simulink model "Mpc_SimMechanics_with_standing"  (R2017b)
settings: Solver=ode45  StartTime=0  StopTime=10  FixedStep=0.0005  EnableMultiTasking=on
InitFcn:
  | isSim = 1;
  | 
  | PreFunctions.CustomInitFcn_with_standing;
  | PreFunctions.simulationInitFcn_with_standing;
undefined symbols (not defined in the file): alpha_x, alpha_y, DiagnosticCodes, DynamicMatrixLibrary, motorPositions, motorVelocities, pelvisPosition, pelvisVelocity, sample_time, X, Y, Z
libraries: sm_lib x170, nesl_utility x75, Contact_Forces_Lib x6, ComponentLibrary x5, xpcrtudplib x2, slrtlib x1
(part 7 of 8)

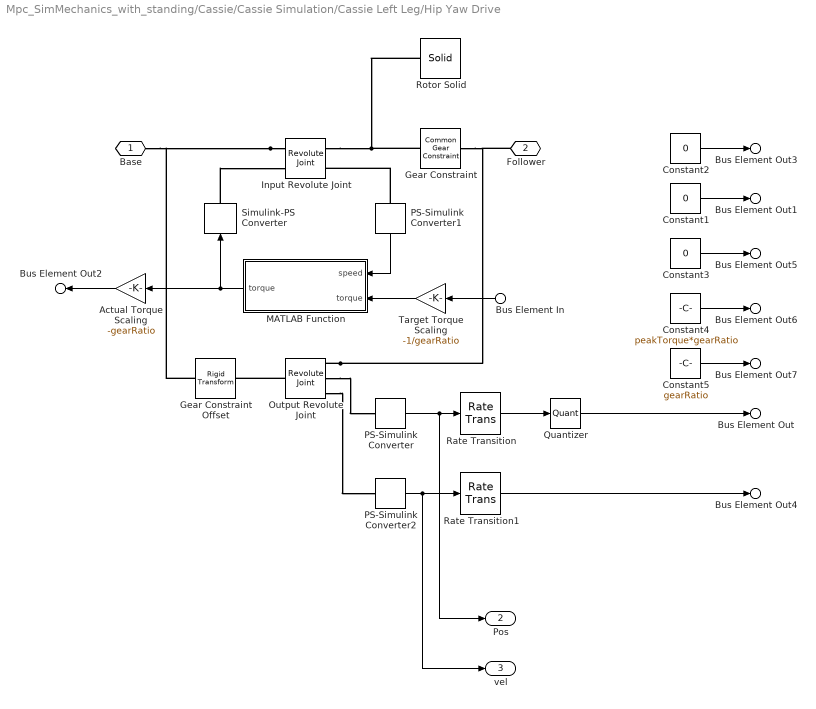
== system Mpc_SimMechanics_with_standing/Cassie/Cassie Simulation/Cassie Left Leg/Hip Yaw Drive ==
  Bus Element In : Inport  PortName=InBus  Element=torque
  Actual Torque Scaling : Gain  Gain=-gearRatio
  Constant1 : Constant  Value=0
  Constant2 : Constant  Value=0  OutDataTypeStr=uint16
  Constant3 : Constant  Value=0
  Constant4 : Constant  Value=peakTorque*gearRatio
  Constant5 : Constant  Value=gearRatio
  Gear Constraint : sm_lib/Gears and Couplings/Gears/Common Gear Constraint  GearType=External  SpecificationType=CenterDistanceRatio  CenterDistance=1e-6  CenterDistanceUnits=m  GearRatio=gearRatio  BaseGearRadius=10.0  BaseGearRadiusUnits=cm  FollGearRadius=10.0  FollGearRadiusUnits=cm  AssemblyGearRotation=Free
      settings: SourceProductName=Simscape Multibody  SourceProductBaseCode=MS
  Gear Constraint Offset : sm_lib/Frames and Transforms/Rigid Transform  TranslationMethod=StandardAxis  TranslationStandardOffset=1e-6  TranslationLengthUnit=m  TranslationStandardAxis=+Y  TranslationCartesianOffset=[0 0 0]  TranslationROffset=0  TranslationROffsetUnits=m  TranslationZOffset=0  TranslationZOffsetUnits=m  TranslationThetaOffset=0  TranslationThetaOffsetUnits=deg  RotationMethod=None  RotationAngleUnits=deg  RotationStandardAxis=+Z  RotationAngle=0.0  RotationArbitraryAxis=[0 0 1]  FollAlignAxisA=+X  BaseAlignAxisA=+Y  FollAlignAxisB=+Y  BaseAlignAxisB=+Z  RotationSequenceAxes=FollowerAxes  RotationSequence=XYX  RotationSequenceAngles=[0 0 0]  RotationSequenceAnglesUnits=deg  RotationMatrix=[1 0 0; 0 1 0; 0 0 1]
  Input Revolute Joint : sm_lib/Joints/Revolute Joint  SenseConstraintForce=off  SenseConstraintForceX=off  SenseConstraintForceY=off  SenseConstraintForceZ=off  SenseConstraintTorque=off  SenseConstraintTorqueX=off  SenseConstraintTorqueY=off  SenseConstraintTorqueZ=off  SenseTotalForce=off  SenseTotalForceX=off  SenseTotalForceY=off  SenseTotalForceZ=off  SenseTotalTorque=off  SenseTotalTorqueX=off  SenseTotalTorqueY=off  SenseTotalTorqueZ=off  CompositeWrenchDir=FollowerOnBase  CompositeWrenchFrame=BaseFrame  EquilibriumPosition=0  EquilibriumPositionUnits=rad  SpringStiffness=0  SpringStiffnessUnits=N*m/rad  DampingCoefficient=0  DampingCoefficientUnits=N*m/(rad/s)  TorqueActuationMode=InputTorque  MotionActuationMode=ComputedMotion  SensePosition=off  SenseVelocity=on  SenseAcceleration=off  SenseTorqueForce=off  PositionTargetSpecify=off  PositionTargetPriority=High  PositionTargetValue=0  PositionTargetValueUnits=deg  VelocityTargetSpecify=off  VelocityTargetPriority=High  VelocityTargetValue=0  VelocityTargetValueUnits=rad/s
  MATLAB Function : MATLAB Function  TreatAsAtomicUnit=on
  Output Revolute Joint : sm_lib/Joints/Revolute Joint  SenseConstraintForce=off  SenseConstraintForceX=off  SenseConstraintForceY=off  SenseConstraintForceZ=off  SenseConstraintTorque=off  SenseConstraintTorqueX=off  SenseConstraintTorqueY=off  SenseConstraintTorqueZ=off  SenseTotalForce=off  SenseTotalForceX=off  SenseTotalForceY=off  SenseTotalForceZ=off  SenseTotalTorque=off  SenseTotalTorqueX=off  SenseTotalTorqueY=off  SenseTotalTorqueZ=off  CompositeWrenchDir=FollowerOnBase  CompositeWrenchFrame=BaseFrame  EquilibriumPosition=0  EquilibriumPositionUnits=rad  SpringStiffness=0  SpringStiffnessUnits=N*m/rad  DampingCoefficient=1  DampingCoefficientUnits=N*m/(rad/s)  TorqueActuationMode=NoTorque  MotionActuationMode=ComputedMotion  SensePosition=on  SenseVelocity=on  SenseAcceleration=off  SenseTorqueForce=off  PositionTargetSpecify=on  PositionTargetPriority=High  PositionTargetValue=initialPosition  PositionTargetValueUnits=rad  VelocityTargetSpecify=on  VelocityTargetPriority=High  VelocityTargetValue=initialVelocity  VelocityTargetValueUnits=rad/s
  PS-Simulink Converter : nesl_utility/PS-Simulink Converter  PhysicalDomain=network_engine_domain  SubClassName=ps_output  LeftPortType=input  RightPortType=output  PseudoPeriodic=off  Frequencies=[]  Unit=rad  AffineConversion=off
  PS-Simulink Converter1 : nesl_utility/PS-Simulink Converter  PhysicalDomain=network_engine_domain  SubClassName=ps_output  LeftPortType=input  RightPortType=output  PseudoPeriodic=off  Frequencies=[]  Unit=rad/s  AffineConversion=off
  PS-Simulink Converter2 : nesl_utility/PS-Simulink Converter  PhysicalDomain=network_engine_domain  SubClassName=ps_output  LeftPortType=input  RightPortType=output  PseudoPeriodic=off  Frequencies=[]  Unit=rad/s  AffineConversion=off
  Quantizer : Quantizer  QuantizationInterval=(2*pi)/(encoderResolution*gearRatio)
  Rate Transition : RateTransition  Deterministic=off  InitialCondition=initialPosition  OutPortSampleTimeOpt=Inherit
  Rate Transition1 : RateTransition  Deterministic=off  InitialCondition=initialPosition  OutPortSampleTimeOpt=Inherit
  Rotor Solid : sm_lib/Body Elements/Solid  InertiaType=Custom  Mass=0  MassUnits=kg  CenterOfMass=[0; 0; 0]  CenterOfMassUnits=m  MomentsOfInertia=[0; 0; rotorInertia]  MomentsOfInertiaUnits=kg*m^2  ProductsOfInertia=[0; 0; 0]  ProductsOfInertiaUnits=kg*m^2  DensityBased=on  Density=1000  DensityUnits=kg/m^3  DoExposeReferenceFrame=on  SerializedFrames=<Frames/>  GraphicType=None  MarkerShape=Sphere  MarkerSize=10  GraphicVisPropType=SimpleVisualProperties  GraphicDiffuseColor=[0.5 0.5 0.5]  GraphicSpecularColor=[0.5 0.5 0.5 1.0]  GraphicAmbientColor=[0.15 0.15 0.15 1.0]  GraphicEmissiveColor=[0.0 0.0 0.0 1.0]  GraphicShininess=75  GraphicOpacity=1.0  GeometryShape=Cylinder  RectangleSize=[1 1]  RectangleSizeUnits=m  BrickDimensions=[1 1 1]  BrickDimensionUnits=m  CylinderRadius=1  CylinderRadiusUnits=m  CylinderLength=1  CylinderLengthUnits=m  SphereRadius=1  SphereRadiusUnits=m  EllipsoidRadii=[1 1 1]  EllipsoidRadiiUnits=m  ExtrusionCrossSection=[1 1; -1 1; -1 -1; 1 -1]  ExtrusionCrossSectionUnits=m  ExtrusionLength=1  ExtrusionLengthUnits=m  PolygonNumSides=3  PolygonOuterRadius=1  PolygonOuterRadiusUnits=m  ExtGeomFileType=STEP  ExtGeomFileUnits=m  RevolutionCrossSection=[1 1; 1 -1; 2 -1; 2 1]  RevolutionCrossSectionUnits=m  RevolutionExtent=Full  RevolutionAngle=180  RevolutionAngleUnits=deg
  Simulink-PS Converter : nesl_utility/Simulink-PS Converter  PhysicalDomain=network_engine_domain  SubClassName=ps_input  LeftPortType=input  RightPortType=output  PseudoPeriodic=off  Frequencies=[]  NoiseDistribution=none  NoiseParameters=[]  Unit=N*m  AffineConversion=off  FilteringAndDerivatives=zero  SimscapeFilterOrder=1  InputFilterTimeConstant=0.001  UdotUserProvided=1
  Target Torque Scaling : Gain  Gain=-1/gearRatio
  Base : PMIOPort  Port=1  Side=Left
  Follower : PMIOPort  Port=2  Side=Right
  Bus Element Out3 : Outport  PortName=OutBus  Element=statusWord
  Bus Element Out : Outport  PortName=OutBus  Element=position
  Bus Element Out4 : Outport  PortName=OutBus  Element=velocity
  Bus Element Out2 : Outport  PortName=OutBus  Element=torque
  Bus Element Out1 : Outport  PortName=OutBus  Element=driveTemperature
  Bus Element Out5 : Outport  PortName=OutBus  Element=dcLinkVoltage
  Bus Element Out6 : Outport  PortName=OutBus  Element=torqueLimit
  Bus Element Out7 : Outport  PortName=OutBus  Element=gearRatio
  Pos : Outport  Port=2
  vel : Outport  Port=3
  wires:
  PS-Simulink Converter2/1 -> vel/1, Rate Transition1/1
  Rate Transition1/1 -> Bus Element Out4/1
  Constant5/1 -> Bus Element Out7/1
  Actual Torque Scaling/1 -> Bus Element Out2/1
  Constant4/1 -> Bus Element Out6/1
  Constant3/1 -> Bus Element Out5/1
  Constant1/1 -> Bus Element Out1/1
  Constant2/1 -> Bus Element Out3/1
  Target Torque Scaling/1 -> MATLAB Function/2("torque ")
  PS-Simulink Converter1/1 -> MATLAB Function/1(speed)
  MATLAB Function/1(torque) -> Simulink-PS Converter/1, Actual Torque Scaling/1
  Bus Element In/1 -> Target Torque Scaling/1
  Quantizer/1 -> Bus Element Out/1
  PS-Simulink Converter/1 -> Pos/1, Rate Transition/1
  Rate Transition/1 -> Quantizer/1
  connections:
  Output Revolute Joint/RConn3 -- PS-Simulink Converter2/LConn1
  Input Revolute Joint/LConn1 -- Base/RConn1 -- Gear Constraint Offset/LConn1
  Simulink-PS Converter/RConn1 -- Input Revolute Joint/LConn2
  PS-Simulink Converter1/LConn1 -- Input Revolute Joint/RConn2
  Rotor Solid/RConn1 -- Gear Constraint/LConn1 -- Input Revolute Joint/RConn1
  Output Revolute Joint/RConn1 -- Follower/RConn1 -- Gear Constraint/RConn1
  Output Revolute Joint/LConn1 -- Gear Constraint Offset/RConn1
  Output Revolute Joint/RConn2 -- PS-Simulink Converter/LConn1

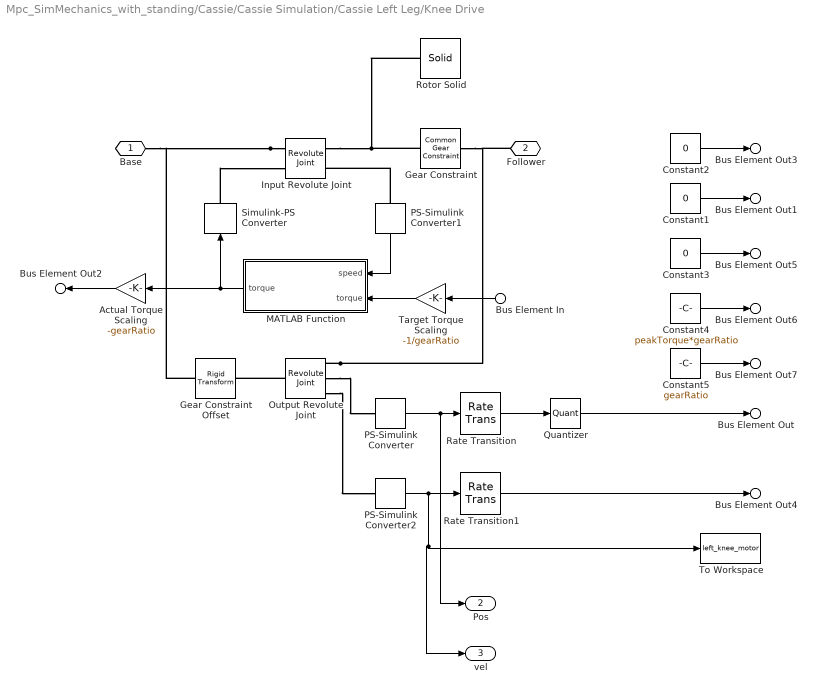
== system Mpc_SimMechanics_with_standing/Cassie/Cassie Simulation/Cassie Left Leg/Knee Drive ==
  Bus Element In : Inport  PortName=InBus  Element=torque
  Actual Torque Scaling : Gain  Gain=-gearRatio
  Constant1 : Constant  Value=0
  Constant2 : Constant  Value=0  OutDataTypeStr=uint16
  Constant3 : Constant  Value=0
  Constant4 : Constant  Value=peakTorque*gearRatio
  Constant5 : Constant  Value=gearRatio
  Gear Constraint : sm_lib/Gears and Couplings/Gears/Common Gear Constraint  GearType=External  SpecificationType=CenterDistanceRatio  CenterDistance=1e-6  CenterDistanceUnits=m  GearRatio=gearRatio  BaseGearRadius=10.0  BaseGearRadiusUnits=cm  FollGearRadius=10.0  FollGearRadiusUnits=cm  AssemblyGearRotation=Free
      settings: SourceProductName=Simscape Multibody  SourceProductBaseCode=MS
  Gear Constraint Offset : sm_lib/Frames and Transforms/Rigid Transform  TranslationMethod=StandardAxis  TranslationStandardOffset=1e-6  TranslationLengthUnit=m  TranslationStandardAxis=+Y  TranslationCartesianOffset=[0 0 0]  TranslationROffset=0  TranslationROffsetUnits=m  TranslationZOffset=0  TranslationZOffsetUnits=m  TranslationThetaOffset=0  TranslationThetaOffsetUnits=deg  RotationMethod=None  RotationAngleUnits=deg  RotationStandardAxis=+Z  RotationAngle=0.0  RotationArbitraryAxis=[0 0 1]  FollAlignAxisA=+X  BaseAlignAxisA=+Y  FollAlignAxisB=+Y  BaseAlignAxisB=+Z  RotationSequenceAxes=FollowerAxes  RotationSequence=XYX  RotationSequenceAngles=[0 0 0]  RotationSequenceAnglesUnits=deg  RotationMatrix=[1 0 0; 0 1 0; 0 0 1]
  Input Revolute Joint : sm_lib/Joints/Revolute Joint  SenseConstraintForce=off  SenseConstraintForceX=off  SenseConstraintForceY=off  SenseConstraintForceZ=off  SenseConstraintTorque=off  SenseConstraintTorqueX=off  SenseConstraintTorqueY=off  SenseConstraintTorqueZ=off  SenseTotalForce=off  SenseTotalForceX=off  SenseTotalForceY=off  SenseTotalForceZ=off  SenseTotalTorque=off  SenseTotalTorqueX=off  SenseTotalTorqueY=off  SenseTotalTorqueZ=off  CompositeWrenchDir=FollowerOnBase  CompositeWrenchFrame=BaseFrame  EquilibriumPosition=0  EquilibriumPositionUnits=rad  SpringStiffness=0  SpringStiffnessUnits=N*m/rad  DampingCoefficient=0  DampingCoefficientUnits=N*m/(rad/s)  TorqueActuationMode=InputTorque  MotionActuationMode=ComputedMotion  SensePosition=off  SenseVelocity=on  SenseAcceleration=off  SenseTorqueForce=off  PositionTargetSpecify=off  PositionTargetPriority=High  PositionTargetValue=0  PositionTargetValueUnits=deg  VelocityTargetSpecify=off  VelocityTargetPriority=High  VelocityTargetValue=0  VelocityTargetValueUnits=rad/s
  MATLAB Function : MATLAB Function  TreatAsAtomicUnit=on
  Output Revolute Joint : sm_lib/Joints/Revolute Joint  SenseConstraintForce=off  SenseConstraintForceX=off  SenseConstraintForceY=off  SenseConstraintForceZ=off  SenseConstraintTorque=off  SenseConstraintTorqueX=off  SenseConstraintTorqueY=off  SenseConstraintTorqueZ=off  SenseTotalForce=off  SenseTotalForceX=off  SenseTotalForceY=off  SenseTotalForceZ=off  SenseTotalTorque=off  SenseTotalTorqueX=off  SenseTotalTorqueY=off  SenseTotalTorqueZ=off  CompositeWrenchDir=FollowerOnBase  CompositeWrenchFrame=BaseFrame  EquilibriumPosition=0  EquilibriumPositionUnits=rad  SpringStiffness=0  SpringStiffnessUnits=N*m/rad  DampingCoefficient=1  DampingCoefficientUnits=N*m/(rad/s)  TorqueActuationMode=NoTorque  MotionActuationMode=ComputedMotion  SensePosition=on  SenseVelocity=on  SenseAcceleration=off  SenseTorqueForce=off  PositionTargetSpecify=on  PositionTargetPriority=High  PositionTargetValue=initialPosition  PositionTargetValueUnits=rad  VelocityTargetSpecify=on  VelocityTargetPriority=High  VelocityTargetValue=initialVelocity  VelocityTargetValueUnits=rad/s
  PS-Simulink Converter : nesl_utility/PS-Simulink Converter  PhysicalDomain=network_engine_domain  SubClassName=ps_output  LeftPortType=input  RightPortType=output  PseudoPeriodic=off  Frequencies=[]  Unit=rad  AffineConversion=off
  PS-Simulink Converter1 : nesl_utility/PS-Simulink Converter  PhysicalDomain=network_engine_domain  SubClassName=ps_output  LeftPortType=input  RightPortType=output  PseudoPeriodic=off  Frequencies=[]  Unit=rad/s  AffineConversion=off
  PS-Simulink Converter2 : nesl_utility/PS-Simulink Converter  PhysicalDomain=network_engine_domain  SubClassName=ps_output  LeftPortType=input  RightPortType=output  PseudoPeriodic=off  Frequencies=[]  Unit=rad/s  AffineConversion=off
  Quantizer : Quantizer  QuantizationInterval=(2*pi)/(encoderResolution*gearRatio)
  Rate Transition : RateTransition  Deterministic=off  InitialCondition=initialPosition  OutPortSampleTimeOpt=Inherit
  Rate Transition1 : RateTransition  Deterministic=off  InitialCondition=initialPosition  OutPortSampleTimeOpt=Inherit
  Rotor Solid : sm_lib/Body Elements/Solid  InertiaType=Custom  Mass=0  MassUnits=kg  CenterOfMass=[0; 0; 0]  CenterOfMassUnits=m  MomentsOfInertia=[0; 0; rotorInertia]  MomentsOfInertiaUnits=kg*m^2  ProductsOfInertia=[0; 0; 0]  ProductsOfInertiaUnits=kg*m^2  DensityBased=on  Density=1000  DensityUnits=kg/m^3  DoExposeReferenceFrame=on  SerializedFrames=<Frames/>  GraphicType=None  MarkerShape=Sphere  MarkerSize=10  GraphicVisPropType=SimpleVisualProperties  GraphicDiffuseColor=[0.5 0.5 0.5]  GraphicSpecularColor=[0.5 0.5 0.5 1.0]  GraphicAmbientColor=[0.15 0.15 0.15 1.0]  GraphicEmissiveColor=[0.0 0.0 0.0 1.0]  GraphicShininess=75  GraphicOpacity=1.0  GeometryShape=Cylinder  RectangleSize=[1 1]  RectangleSizeUnits=m  BrickDimensions=[1 1 1]  BrickDimensionUnits=m  CylinderRadius=1  CylinderRadiusUnits=m  CylinderLength=1  CylinderLengthUnits=m  SphereRadius=1  SphereRadiusUnits=m  EllipsoidRadii=[1 1 1]  EllipsoidRadiiUnits=m  ExtrusionCrossSection=[1 1; -1 1; -1 -1; 1 -1]  ExtrusionCrossSectionUnits=m  ExtrusionLength=1  ExtrusionLengthUnits=m  PolygonNumSides=3  PolygonOuterRadius=1  PolygonOuterRadiusUnits=m  ExtGeomFileType=STEP  ExtGeomFileUnits=m  RevolutionCrossSection=[1 1; 1 -1; 2 -1; 2 1]  RevolutionCrossSectionUnits=m  RevolutionExtent=Full  RevolutionAngle=180  RevolutionAngleUnits=deg
  Simulink-PS Converter : nesl_utility/Simulink-PS Converter  PhysicalDomain=network_engine_domain  SubClassName=ps_input  LeftPortType=input  RightPortType=output  PseudoPeriodic=off  Frequencies=[]  NoiseDistribution=none  NoiseParameters=[]  Unit=N*m  AffineConversion=off  FilteringAndDerivatives=zero  SimscapeFilterOrder=1  InputFilterTimeConstant=0.001  UdotUserProvided=1
  Target Torque Scaling : Gain  Gain=-1/gearRatio
  To Workspace : ToWorkspace  VariableName=left_knee_motor  SaveFormat=Timeseries  SampleTime=-1
  Base : PMIOPort  Port=1  Side=Left
  Follower : PMIOPort  Port=2  Side=Right
  Bus Element Out3 : Outport  PortName=OutBus  Element=statusWord
  Bus Element Out : Outport  PortName=OutBus  Element=position
  Bus Element Out4 : Outport  PortName=OutBus  Element=velocity
  Bus Element Out2 : Outport  PortName=OutBus  Element=torque
  Bus Element Out1 : Outport  PortName=OutBus  Element=driveTemperature
  Bus Element Out5 : Outport  PortName=OutBus  Element=dcLinkVoltage
  Bus Element Out6 : Outport  PortName=OutBus  Element=torqueLimit
  Bus Element Out7 : Outport  PortName=OutBus  Element=gearRatio
  Pos : Outport  Port=2
  vel : Outport  Port=3
  wires:
  PS-Simulink Converter2/1 -> vel/1, To Workspace/1, Rate Transition1/1
  Rate Transition1/1 -> Bus Element Out4/1
  Constant5/1 -> Bus Element Out7/1
  Actual Torque Scaling/1 -> Bus Element Out2/1
  Constant4/1 -> Bus Element Out6/1
  Constant3/1 -> Bus Element Out5/1
  Constant1/1 -> Bus Element Out1/1
  Constant2/1 -> Bus Element Out3/1
  Target Torque Scaling/1 -> MATLAB Function/2("torque ")
  PS-Simulink Converter1/1 -> MATLAB Function/1(speed)
  MATLAB Function/1(torque) -> Simulink-PS Converter/1, Actual Torque Scaling/1
  Bus Element In/1 -> Target Torque Scaling/1
  Quantizer/1 -> Bus Element Out/1
  PS-Simulink Converter/1 -> Pos/1, Rate Transition/1
  Rate Transition/1 -> Quantizer/1
  connections:
  Output Revolute Joint/RConn3 -- PS-Simulink Converter2/LConn1
  Input Revolute Joint/LConn1 -- Base/RConn1 -- Gear Constraint Offset/LConn1
  Simulink-PS Converter/RConn1 -- Input Revolute Joint/LConn2
  PS-Simulink Converter1/LConn1 -- Input Revolute Joint/RConn2
  Rotor Solid/RConn1 -- Gear Constraint/LConn1 -- Input Revolute Joint/RConn1
  Output Revolute Joint/RConn1 -- Follower/RConn1 -- Gear Constraint/RConn1
  Output Revolute Joint/LConn1 -- Gear Constraint Offset/RConn1
  Output Revolute Joint/RConn2 -- PS-Simulink Converter/LConn1

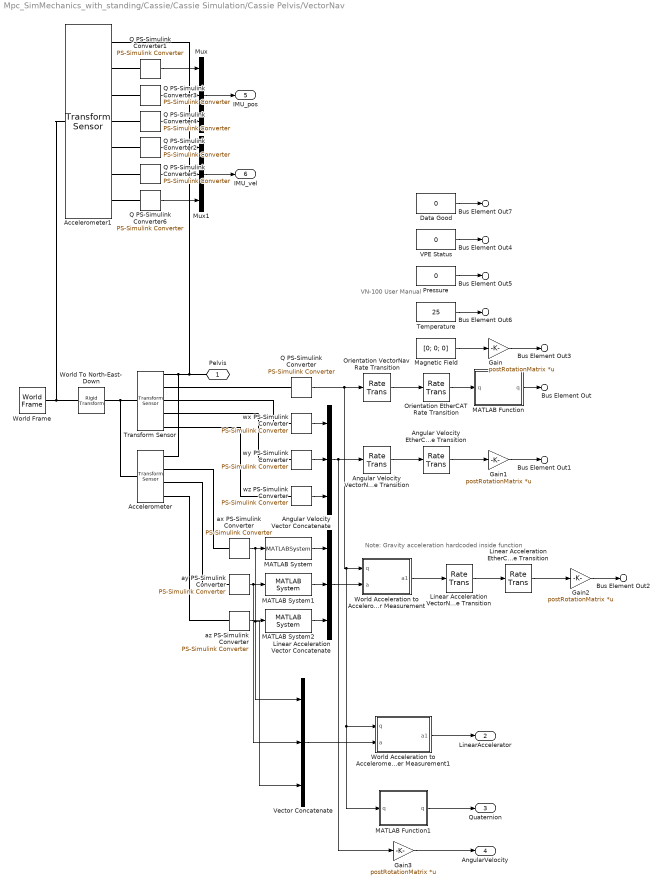
== system Mpc_SimMechanics_with_standing/Cassie/Cassie Simulation/Cassie Pelvis/VectorNav ==
  note: VN-100 User Manual
  note: Note: Gravity acceleration hardcoded inside function
  Accelerometer : sm_lib/Frames and Transforms/Transform Sensor  MeasurementFrame=Base  SenseAngle=off  SenseAxis=off  SenseAngle1=off  SenseAngle2=off  SenseAngle3=off  SenseQ=off  SenseR=off  SenseOmegaX=off  SenseOmegaY=off  SenseOmegaZ=off  SenseOmega1=off  SenseOmega2=off  SenseOmega3=off  SenseQDot=off  SenseRDot=off  SenseAlphaX=off  SenseAlphaY=off  SenseAlphaZ=off  SenseAlpha1=off  SenseAlpha2=off  SenseAlpha3=off  SenseQDDot=off  SenseRDDot=off  SenseX=off  SenseY=off  SenseZ=off  SenseRad=off  SenseAzim=off  SenseDist=off  SenseInc=off  SenseXDot=off  SenseYDot=off  SenseZDot=off  SenseRadDot=off  SenseAzimDot=off  SenseDistDot=off  SenseIncDot=off  SenseXDDot=on  SenseYDDot=on  SenseZDDot=on  SenseRadDDot=off  SenseAzimDDot=off  SenseDistDDot=off  SenseIncDDot=off
  Accelerometer1 : sm_lib/Frames and Transforms/Transform Sensor  MeasurementFrame=Base  SenseAngle=off  SenseAxis=off  SenseAngle1=off  SenseAngle2=off  SenseAngle3=off  SenseQ=off  SenseR=off  SenseOmegaX=off  SenseOmegaY=off  SenseOmegaZ=off  SenseOmega1=off  SenseOmega2=off  SenseOmega3=off  SenseQDot=off  SenseRDot=off  SenseAlphaX=off  SenseAlphaY=off  SenseAlphaZ=off  SenseAlpha1=off  SenseAlpha2=off  SenseAlpha3=off  SenseQDDot=off  SenseRDDot=off  SenseX=on  SenseY=on  SenseZ=on  SenseRad=off  SenseAzim=off  SenseDist=off  SenseInc=off  SenseXDot=on  SenseYDot=on  SenseZDot=on  SenseRadDot=off  SenseAzimDot=off  SenseDistDot=off  SenseIncDot=off  SenseXDDot=off  SenseYDDot=off  SenseZDDot=off  SenseRadDDot=off  SenseAzimDDot=off  SenseDistDDot=off  SenseIncDDot=off
  Angular Velocity EtherCAT Rate Transition : RateTransition  Deterministic=off  OutPortSampleTimeOpt=Inherit
  Angular Velocity Vector Concatenate : Concatenate  NumInputs=3
  Angular Velocity VectorNav Rate Transition : RateTransition  Deterministic=off  OutPortSampleTime=VectorNavModule.sampleTime
  Data Good : Constant  Value=0  OutDataTypeStr=boolean
  Gain{,1..3} (4 alike) : Gain  Gain=postRotationMatrix  Multiplication=Matrix(K*u)
  Linear Acceleration EtherCAT Rate Transition : RateTransition  Deterministic=off  InitialCondition=[0; 0; 0]  OutPortSampleTimeOpt=Inherit
  Linear Acceleration Vector Concatenate : Concatenate  NumInputs=3
  Linear Acceleration VectorNav Rate Transition : RateTransition  Deterministic=off  InitialCondition=[0; 0; 0]  OutPortSampleTime=VectorNavModule.sampleTime
  MATLAB Function : MATLAB Function  TreatAsAtomicUnit=on
  MATLAB Function1 : MATLAB Function  TreatAsAtomicUnit=on
  MATLAB System : MATLABSystem  System=FilterSystem  a=[1 -0.8]  b=0.2  SimulateUsing=Code generation
      mask Type: FilterSystem
      mask Display: disp('Filter');
  MATLAB System1 : ComponentLibrary/Simulation/VectorNav/MATLAB System  a=[1 -0.8]  b=0.2  SimulateUsing=Code generation
  MATLAB System2 : ComponentLibrary/Simulation/VectorNav/MATLAB System  a=[1 -0.8]  b=0.2  SimulateUsing=Code generation
  Magnetic Field : Constant  Value=[0; 0; 0]
  Mux : Mux  Inputs=3
  Mux1 : Mux  Inputs=3
  Orientation EtherCAT Rate Transition : RateTransition  Deterministic=off  InitialCondition=[0; 0; 0; 1]  OutPortSampleTimeOpt=Inherit
  Orientation VectorNav Rate Transition : RateTransition  Deterministic=off  InitialCondition=[0; 0; 0; 1]  OutPortSampleTime=VectorNavModule.sampleTime
  Pressure : Constant  Value=0
  Q PS-Simulink Converter : nesl_utility/PS-Simulink Converter  PhysicalDomain=network_engine_domain  SubClassName=ps_output  LeftPortType=input  RightPortType=output  PseudoPeriodic=off  Frequencies=[]  Unit=1  AffineConversion=off
  Q PS-Simulink Converter1 : nesl_utility/PS-Simulink Converter  PhysicalDomain=network_engine_domain  SubClassName=ps_output  LeftPortType=input  RightPortType=output  PseudoPeriodic=off  Frequencies=[]  Unit=m  AffineConversion=off
  Q PS-Simulink Converter2 : nesl_utility/PS-Simulink Converter  PhysicalDomain=network_engine_domain  SubClassName=ps_output  LeftPortType=input  RightPortType=output  PseudoPeriodic=off  Frequencies=[]  Unit=m/s  AffineConversion=off
  Q PS-Simulink Converter3 : nesl_utility/PS-Simulink Converter  PhysicalDomain=network_engine_domain  SubClassName=ps_output  LeftPortType=input  RightPortType=output  PseudoPeriodic=off  Frequencies=[]  Unit=m  AffineConversion=off
  Q PS-Simulink Converter4 : nesl_utility/PS-Simulink Converter  PhysicalDomain=network_engine_domain  SubClassName=ps_output  LeftPortType=input  RightPortType=output  PseudoPeriodic=off  Frequencies=[]  Unit=m  AffineConversion=off
  Q PS-Simulink Converter5 : nesl_utility/PS-Simulink Converter  PhysicalDomain=network_engine_domain  SubClassName=ps_output  LeftPortType=input  RightPortType=output  PseudoPeriodic=off  Frequencies=[]  Unit=m/s  AffineConversion=off
  Q PS-Simulink Converter6 : nesl_utility/PS-Simulink Converter  PhysicalDomain=network_engine_domain  SubClassName=ps_output  LeftPortType=input  RightPortType=output  PseudoPeriodic=off  Frequencies=[]  Unit=m/s  AffineConversion=off
  Temperature : Constant  Value=25
  Transform Sensor : sm_lib/Frames and Transforms/Transform Sensor  MeasurementFrame=Follower  SenseAngle=off  SenseAxis=off  SenseAngle1=off  SenseAngle2=off  SenseAngle3=off  SenseQ=on  SenseR=off  SenseOmegaX=on  SenseOmegaY=on  SenseOmegaZ=on  SenseOmega1=off  SenseOmega2=off  SenseOmega3=off  SenseQDot=off  SenseRDot=off  SenseAlphaX=off  SenseAlphaY=off  SenseAlphaZ=off  SenseAlpha1=off  SenseAlpha2=off  SenseAlpha3=off  SenseQDDot=off  SenseRDDot=off  SenseX=off  SenseY=off  SenseZ=off  SenseRad=off  SenseAzim=off  SenseDist=off  SenseInc=off  SenseXDot=off  SenseYDot=off  SenseZDot=off  SenseRadDot=off  SenseAzimDot=off  SenseDistDot=off  SenseIncDot=off  SenseXDDot=off  SenseYDDot=off  SenseZDDot=off  SenseRadDDot=off  SenseAzimDDot=off  SenseDistDDot=off  SenseIncDDot=off
  VPE Status : Constant  Value=0  OutDataTypeStr=uint16
  Vector Concatenate : Concatenate  NumInputs=3
  World Acceleration to Accelerometer Measurement : MATLAB Function  TreatAsAtomicUnit=on
  World Acceleration to Accelerometer Measurement1 : MATLAB Function  TreatAsAtomicUnit=on
  World Frame : sm_lib/Frames and Transforms/World Frame
  World To North-East-Down : sm_lib/Frames and Transforms/Rigid Transform  TranslationMethod=None  TranslationStandardOffset=0  TranslationLengthUnit=m  TranslationStandardAxis=+Z  TranslationCartesianOffset=[0 0 0]  TranslationROffset=0  TranslationROffsetUnits=m  TranslationZOffset=0  TranslationZOffsetUnits=m  TranslationThetaOffset=0  TranslationThetaOffsetUnits=deg  RotationMethod=StandardAxis  RotationAngleUnits=deg  RotationStandardAxis=+X  RotationAngle=180  RotationArbitraryAxis=[0 0 1]  FollAlignAxisA=+X  BaseAlignAxisA=+Y  FollAlignAxisB=+Y  BaseAlignAxisB=+Z  RotationSequenceAxes=FollowerAxes  RotationSequence=XYX  RotationSequenceAngles=[0 0 0]  RotationSequenceAnglesUnits=deg  RotationMatrix=[1 0 0; 0 1 0; 0 0 1]
  ax PS-Simulink Converter : nesl_utility/PS-Simulink Converter  PhysicalDomain=network_engine_domain  SubClassName=ps_output  LeftPortType=input  RightPortType=output  PseudoPeriodic=off  Frequencies=[]  Unit=m/s/s  AffineConversion=off
  ay PS-Simulink Converter : nesl_utility/PS-Simulink Converter  PhysicalDomain=network_engine_domain  SubClassName=ps_output  LeftPortType=input  RightPortType=output  PseudoPeriodic=off  Frequencies=[]  Unit=m/s/s  AffineConversion=off
  az PS-Simulink Converter : nesl_utility/PS-Simulink Converter  PhysicalDomain=network_engine_domain  SubClassName=ps_output  LeftPortType=input  RightPortType=output  PseudoPeriodic=off  Frequencies=[]  Unit=m/s/s  AffineConversion=off
  wx PS-Simulink Converter : nesl_utility/PS-Simulink Converter  PhysicalDomain=network_engine_domain  SubClassName=ps_output  LeftPortType=input  RightPortType=output  PseudoPeriodic=off  Frequencies=[]  Unit=1  AffineConversion=off
  wy PS-Simulink Converter : nesl_utility/PS-Simulink Converter  PhysicalDomain=network_engine_domain  SubClassName=ps_output  LeftPortType=input  RightPortType=output  PseudoPeriodic=off  Frequencies=[]  Unit=1  AffineConversion=off
  wz PS-Simulink Converter : nesl_utility/PS-Simulink Converter  PhysicalDomain=network_engine_domain  SubClassName=ps_output  LeftPortType=input  RightPortType=output  PseudoPeriodic=off  Frequencies=[]  Unit=1  AffineConversion=off
  Pelvis : PMIOPort  Port=1  Side=Left
  Bus Element Out7 : Outport  PortName=OutBus  Element=dataGood
  Bus Element Out4 : Outport  PortName=OutBus  Element=vpeStatus
  Bus Element Out5 : Outport  PortName=OutBus  Element=pressure
  Bus Element Out6 : Outport  PortName=OutBus  Element=temperature
  Bus Element Out3 : Outport  PortName=OutBus  Element=magneticField
  Bus Element Out1 : Outport  PortName=OutBus  Element=angularVelocity
  Bus Element Out2 : Outport  PortName=OutBus  Element=linearAcceleration
  Bus Element Out : Outport  PortName=OutBus  Element=orientation
  LinearAccelerator : Outport  Port=2
  Quaternion : Outport  Port=3
  AngularVelocity : Outport  Port=4
  IMU_pos : Outport  Port=5
  IMU_vel : Outport  Port=6
  wires:
  Linear Acceleration Vector Concatenate/1 -> World Acceleration to Accelerometer Measurement/2(a)
  World Acceleration to Accelerometer Measurement/1(a1) -> Linear Acceleration VectorNav Rate Transition/1
  Gain2/1 -> Bus Element Out2/1
  MATLAB System2/1 -> Linear Acceleration Vector Concatenate/3
  MATLAB System1/1 -> Linear Acceleration Vector Concatenate/2
  MATLAB System/1 -> Linear Acceleration Vector Concatenate/1
  MATLAB Function/1(q) -> Bus Element Out/1
  Gain1/1 -> Bus Element Out1/1
  Gain/1 -> Bus Element Out3/1
  Pressure/1 -> Bus Element Out5/1
  Angular Velocity Vector Concatenate/1 -> Gain3/1, Angular Velocity VectorNav Rate Transition/1
  Magnetic Field/1 -> Gain/1
  ay PS-Simulink Converter/1 -> Vector Concatenate/2, MATLAB System1/1
  Data Good/1 -> Bus Element Out7/1
  Linear Acceleration VectorNav Rate Transition/1 -> Linear Acceleration EtherCAT Rate Transition/1
  Linear Acceleration EtherCAT Rate Transition/1 -> Gain2/1
  Orientation VectorNav Rate Transition/1 -> Orientation EtherCAT Rate Transition/1
  Angular Velocity EtherCAT Rate Transition/1 -> Gain1/1
  wy PS-Simulink Converter/1 -> Angular Velocity Vector Concatenate/2
  Temperature/1 -> Bus Element Out6/1
  Q PS-Simulink Converter/1 -> Orientation VectorNav Rate Transition/1, MATLAB Function1/1("q "), World Acceleration to Accelerometer Measurement1/1(q), World Acceleration to Accelerometer Measurement/1(q)
  Orientation EtherCAT Rate Transition/1 -> MATLAB Function/1("q ")
  VPE Status/1 -> Bus Element Out4/1
  ax PS-Simulink Converter/1 -> Vector Concatenate/3, Vector Concatenate/1, MATLAB System/1
  wx PS-Simulink Converter/1 -> Angular Velocity Vector Concatenate/1
  az PS-Simulink Converter/1 -> MATLAB System2/1
  wz PS-Simulink Converter/1 -> Angular Velocity Vector Concatenate/3
  Angular Velocity VectorNav Rate Transition/1 -> Angular Velocity EtherCAT Rate Transition/1
  Vector Concatenate/1 -> World Acceleration to Accelerometer Measurement1/2(a)
  World Acceleration to Accelerometer Measurement1/1(a1) -> LinearAccelerator/1
  MATLAB Function1/1(q) -> Quaternion/1
  Gain3/1 -> AngularVelocity/1
  Q PS-Simulink Converter1/1 -> Mux/1
  Q PS-Simulink Converter3/1 -> Mux/2
  Q PS-Simulink Converter4/1 -> Mux/3
  Q PS-Simulink Converter2/1 -> Mux1/1
  Q PS-Simulink Converter5/1 -> Mux1/2
  Q PS-Simulink Converter6/1 -> Mux1/3
  Mux1/1 -> IMU_vel/1
  Mux/1 -> IMU_pos/1
  connections:
  wz PS-Simulink Converter/LConn1 -- Transform Sensor/RConn5
  Transform Sensor/RConn3 -- wx PS-Simulink Converter/LConn1
  Accelerometer/RConn4 -- az PS-Simulink Converter/LConn1
  Accelerometer/RConn1 -- Accelerometer1/RConn1 -- Pelvis/RConn1 -- Transform Sensor/RConn1
  Accelerometer/RConn2 -- ax PS-Simulink Converter/LConn1
  Q PS-Simulink Converter/LConn1 -- Transform Sensor/RConn2
  World Frame/RConn1 -- Accelerometer1/LConn1 -- World To North-East-Down/LConn1
  Accelerometer/RConn3 -- ay PS-Simulink Converter/LConn1
  Transform Sensor/LConn1 -- Accelerometer/LConn1 -- World To North-East-Down/RConn1
  Transform Sensor/RConn4 -- wy PS-Simulink Converter/LConn1
  Q PS-Simulink Converter1/LConn1 -- Accelerometer1/RConn2
  Q PS-Simulink Converter3/LConn1 -- Accelerometer1/RConn3
  Q PS-Simulink Converter4/LConn1 -- Accelerometer1/RConn4
  Q PS-Simulink Converter2/LConn1 -- Accelerometer1/RConn5
  Q PS-Simulink Converter5/LConn1 -- Accelerometer1/RConn6
  Q PS-Simulink Converter6/LConn1 -- Accelerometer1/RConn7

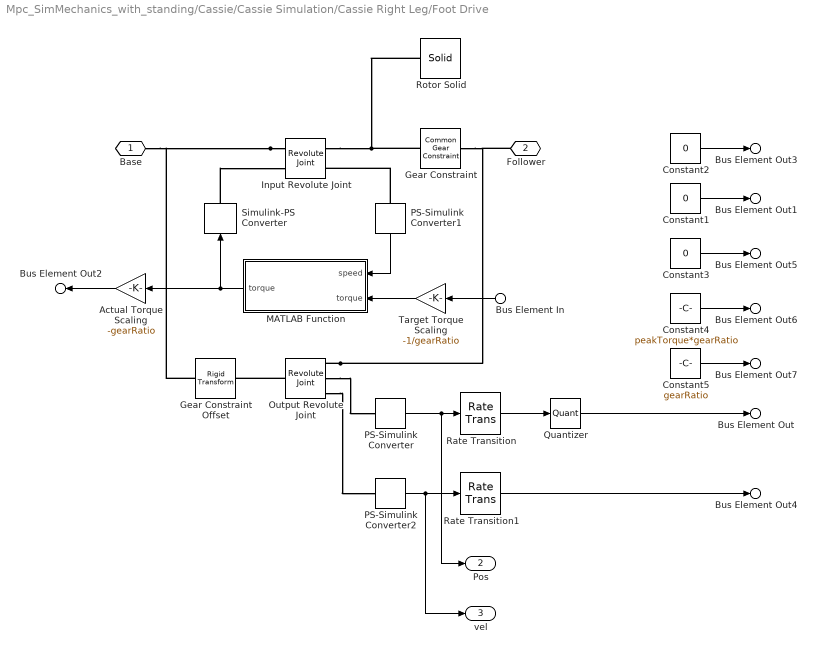
== system Mpc_SimMechanics_with_standing/Cassie/Cassie Simulation/Cassie Right Leg/Foot Drive ==
  Bus Element In : Inport  PortName=InBus  Element=torque
  Actual Torque Scaling : Gain  Gain=-gearRatio
  Constant1 : Constant  Value=0
  Constant2 : Constant  Value=0  OutDataTypeStr=uint16
  Constant3 : Constant  Value=0
  Constant4 : Constant  Value=peakTorque*gearRatio
  Constant5 : Constant  Value=gearRatio
  Gear Constraint : sm_lib/Gears and Couplings/Gears/Common Gear Constraint  GearType=External  SpecificationType=CenterDistanceRatio  CenterDistance=1e-6  CenterDistanceUnits=m  GearRatio=gearRatio  BaseGearRadius=10.0  BaseGearRadiusUnits=cm  FollGearRadius=10.0  FollGearRadiusUnits=cm  AssemblyGearRotation=Free
      settings: SourceProductName=Simscape Multibody  SourceProductBaseCode=MS
  Gear Constraint Offset : sm_lib/Frames and Transforms/Rigid Transform  TranslationMethod=StandardAxis  TranslationStandardOffset=1e-6  TranslationLengthUnit=m  TranslationStandardAxis=+Y  TranslationCartesianOffset=[0 0 0]  TranslationROffset=0  TranslationROffsetUnits=m  TranslationZOffset=0  TranslationZOffsetUnits=m  TranslationThetaOffset=0  TranslationThetaOffsetUnits=deg  RotationMethod=None  RotationAngleUnits=deg  RotationStandardAxis=+Z  RotationAngle=0.0  RotationArbitraryAxis=[0 0 1]  FollAlignAxisA=+X  BaseAlignAxisA=+Y  FollAlignAxisB=+Y  BaseAlignAxisB=+Z  RotationSequenceAxes=FollowerAxes  RotationSequence=XYX  RotationSequenceAngles=[0 0 0]  RotationSequenceAnglesUnits=deg  RotationMatrix=[1 0 0; 0 1 0; 0 0 1]
  Input Revolute Joint : sm_lib/Joints/Revolute Joint  SenseConstraintForce=off  SenseConstraintForceX=off  SenseConstraintForceY=off  SenseConstraintForceZ=off  SenseConstraintTorque=off  SenseConstraintTorqueX=off  SenseConstraintTorqueY=off  SenseConstraintTorqueZ=off  SenseTotalForce=off  SenseTotalForceX=off  SenseTotalForceY=off  SenseTotalForceZ=off  SenseTotalTorque=off  SenseTotalTorqueX=off  SenseTotalTorqueY=off  SenseTotalTorqueZ=off  CompositeWrenchDir=FollowerOnBase  CompositeWrenchFrame=BaseFrame  EquilibriumPosition=0  EquilibriumPositionUnits=rad  SpringStiffness=0  SpringStiffnessUnits=N*m/rad  DampingCoefficient=0  DampingCoefficientUnits=N*m/(rad/s)  TorqueActuationMode=InputTorque  MotionActuationMode=ComputedMotion  SensePosition=off  SenseVelocity=on  SenseAcceleration=off  SenseTorqueForce=off  PositionTargetSpecify=off  PositionTargetPriority=High  PositionTargetValue=0  PositionTargetValueUnits=deg  VelocityTargetSpecify=off  VelocityTargetPriority=High  VelocityTargetValue=0  VelocityTargetValueUnits=rad/s
  MATLAB Function : MATLAB Function  TreatAsAtomicUnit=on
  Output Revolute Joint : sm_lib/Joints/Revolute Joint  SenseConstraintForce=off  SenseConstraintForceX=off  SenseConstraintForceY=off  SenseConstraintForceZ=off  SenseConstraintTorque=off  SenseConstraintTorqueX=off  SenseConstraintTorqueY=off  SenseConstraintTorqueZ=off  SenseTotalForce=off  SenseTotalForceX=off  SenseTotalForceY=off  SenseTotalForceZ=off  SenseTotalTorque=off  SenseTotalTorqueX=off  SenseTotalTorqueY=off  SenseTotalTorqueZ=off  CompositeWrenchDir=FollowerOnBase  CompositeWrenchFrame=BaseFrame  EquilibriumPosition=0  EquilibriumPositionUnits=rad  SpringStiffness=0  SpringStiffnessUnits=N*m/rad  DampingCoefficient=0  DampingCoefficientUnits=N*m/(rad/s)  TorqueActuationMode=NoTorque  MotionActuationMode=ComputedMotion  SensePosition=on  SenseVelocity=on  SenseAcceleration=off  SenseTorqueForce=off  PositionTargetSpecify=on  PositionTargetPriority=High  PositionTargetValue=initialPosition  PositionTargetValueUnits=rad  VelocityTargetSpecify=on  VelocityTargetPriority=High  VelocityTargetValue=initialVelocity  VelocityTargetValueUnits=rad/s
  PS-Simulink Converter : nesl_utility/PS-Simulink Converter  PhysicalDomain=network_engine_domain  SubClassName=ps_output  LeftPortType=input  RightPortType=output  PseudoPeriodic=off  Frequencies=[]  Unit=rad  AffineConversion=off
  PS-Simulink Converter1 : nesl_utility/PS-Simulink Converter  PhysicalDomain=network_engine_domain  SubClassName=ps_output  LeftPortType=input  RightPortType=output  PseudoPeriodic=off  Frequencies=[]  Unit=rad/s  AffineConversion=off
  PS-Simulink Converter2 : nesl_utility/PS-Simulink Converter  PhysicalDomain=network_engine_domain  SubClassName=ps_output  LeftPortType=input  RightPortType=output  PseudoPeriodic=off  Frequencies=[]  Unit=rad/s  AffineConversion=off
  Quantizer : Quantizer  QuantizationInterval=(2*pi)/(encoderResolution*gearRatio)
  Rate Transition : RateTransition  Deterministic=off  InitialCondition=initialPosition  OutPortSampleTimeOpt=Inherit
  Rate Transition1 : RateTransition  Deterministic=off  InitialCondition=initialPosition  OutPortSampleTimeOpt=Inherit
  Rotor Solid : sm_lib/Body Elements/Solid  InertiaType=Custom  Mass=0  MassUnits=kg  CenterOfMass=[0; 0; 0]  CenterOfMassUnits=m  MomentsOfInertia=[0; 0; rotorInertia]  MomentsOfInertiaUnits=kg*m^2  ProductsOfInertia=[0; 0; 0]  ProductsOfInertiaUnits=kg*m^2  DensityBased=on  Density=1000  DensityUnits=kg/m^3  DoExposeReferenceFrame=on  SerializedFrames=<Frames/>  GraphicType=None  MarkerShape=Sphere  MarkerSize=10  GraphicVisPropType=SimpleVisualProperties  GraphicDiffuseColor=[0.5 0.5 0.5]  GraphicSpecularColor=[0.5 0.5 0.5 1.0]  GraphicAmbientColor=[0.15 0.15 0.15 1.0]  GraphicEmissiveColor=[0.0 0.0 0.0 1.0]  GraphicShininess=75  GraphicOpacity=1.0  GeometryShape=Cylinder  RectangleSize=[1 1]  RectangleSizeUnits=m  BrickDimensions=[1 1 1]  BrickDimensionUnits=m  CylinderRadius=1  CylinderRadiusUnits=m  CylinderLength=1  CylinderLengthUnits=m  SphereRadius=1  SphereRadiusUnits=m  EllipsoidRadii=[1 1 1]  EllipsoidRadiiUnits=m  ExtrusionCrossSection=[1 1; -1 1; -1 -1; 1 -1]  ExtrusionCrossSectionUnits=m  ExtrusionLength=1  ExtrusionLengthUnits=m  PolygonNumSides=3  PolygonOuterRadius=1  PolygonOuterRadiusUnits=m  ExtGeomFileType=STEP  ExtGeomFileUnits=m  RevolutionCrossSection=[1 1; 1 -1; 2 -1; 2 1]  RevolutionCrossSectionUnits=m  RevolutionExtent=Full  RevolutionAngle=180  RevolutionAngleUnits=deg
  Simulink-PS Converter : nesl_utility/Simulink-PS Converter  PhysicalDomain=network_engine_domain  SubClassName=ps_input  LeftPortType=input  RightPortType=output  PseudoPeriodic=off  Frequencies=[]  NoiseDistribution=none  NoiseParameters=[]  Unit=N*m  AffineConversion=off  FilteringAndDerivatives=zero  SimscapeFilterOrder=1  InputFilterTimeConstant=0.001  UdotUserProvided=1
  Target Torque Scaling : Gain  Gain=-1/gearRatio
  Base : PMIOPort  Port=1  Side=Left
  Follower : PMIOPort  Port=2  Side=Right
  Bus Element Out3 : Outport  PortName=OutBus  Element=statusWord
  Bus Element Out : Outport  PortName=OutBus  Element=position
  Bus Element Out4 : Outport  PortName=OutBus  Element=velocity
  Bus Element Out2 : Outport  PortName=OutBus  Element=torque
  Bus Element Out1 : Outport  PortName=OutBus  Element=driveTemperature
  Bus Element Out5 : Outport  PortName=OutBus  Element=dcLinkVoltage
  Bus Element Out6 : Outport  PortName=OutBus  Element=torqueLimit
  Bus Element Out7 : Outport  PortName=OutBus  Element=gearRatio
  Pos : Outport  Port=2
  vel : Outport  Port=3
  wires:
  PS-Simulink Converter2/1 -> vel/1, Rate Transition1/1
  Rate Transition1/1 -> Bus Element Out4/1
  Constant5/1 -> Bus Element Out7/1
  Actual Torque Scaling/1 -> Bus Element Out2/1
  Constant4/1 -> Bus Element Out6/1
  Constant3/1 -> Bus Element Out5/1
  Constant1/1 -> Bus Element Out1/1
  Constant2/1 -> Bus Element Out3/1
  Target Torque Scaling/1 -> MATLAB Function/2("torque ")
  PS-Simulink Converter1/1 -> MATLAB Function/1(speed)
  MATLAB Function/1(torque) -> Simulink-PS Converter/1, Actual Torque Scaling/1
  Bus Element In/1 -> Target Torque Scaling/1
  Quantizer/1 -> Bus Element Out/1
  PS-Simulink Converter/1 -> Pos/1, Rate Transition/1
  Rate Transition/1 -> Quantizer/1
  connections:
  Output Revolute Joint/RConn3 -- PS-Simulink Converter2/LConn1
  Input Revolute Joint/LConn1 -- Base/RConn1 -- Gear Constraint Offset/LConn1
  Simulink-PS Converter/RConn1 -- Input Revolute Joint/LConn2
  PS-Simulink Converter1/LConn1 -- Input Revolute Joint/RConn2
  Rotor Solid/RConn1 -- Gear Constraint/LConn1 -- Input Revolute Joint/RConn1
  Output Revolute Joint/RConn1 -- Follower/RConn1 -- Gear Constraint/RConn1
  Output Revolute Joint/LConn1 -- Gear Constraint Offset/RConn1
  Output Revolute Joint/RConn2 -- PS-Simulink Converter/LConn1

== system Mpc_SimMechanics_with_standing/Cassie/Cassie Simulation/Cassie Right Leg/Hip Pitch Drive ==
  Bus Element In : Inport  PortName=InBus  Element=torque
  Actual Torque Scaling : Gain  Gain=-gearRatio
  Constant1 : Constant  Value=0
  Constant2 : Constant  Value=0  OutDataTypeStr=uint16
  Constant3 : Constant  Value=0
  Constant4 : Constant  Value=peakTorque*gearRatio
  Constant5 : Constant  Value=gearRatio
  Gear Constraint : sm_lib/Gears and Couplings/Gears/Common Gear Constraint  GearType=External  SpecificationType=CenterDistanceRatio  CenterDistance=1e-6  CenterDistanceUnits=m  GearRatio=gearRatio  BaseGearRadius=10.0  BaseGearRadiusUnits=cm  FollGearRadius=10.0  FollGearRadiusUnits=cm  AssemblyGearRotation=Free
      settings: SourceProductName=Simscape Multibody  SourceProductBaseCode=MS
  Gear Constraint Offset : sm_lib/Frames and Transforms/Rigid Transform  TranslationMethod=StandardAxis  TranslationStandardOffset=1e-6  TranslationLengthUnit=m  TranslationStandardAxis=+Y  TranslationCartesianOffset=[0 0 0]  TranslationROffset=0  TranslationROffsetUnits=m  TranslationZOffset=0  TranslationZOffsetUnits=m  TranslationThetaOffset=0  TranslationThetaOffsetUnits=deg  RotationMethod=None  RotationAngleUnits=deg  RotationStandardAxis=+Z  RotationAngle=0.0  RotationArbitraryAxis=[0 0 1]  FollAlignAxisA=+X  BaseAlignAxisA=+Y  FollAlignAxisB=+Y  BaseAlignAxisB=+Z  RotationSequenceAxes=FollowerAxes  RotationSequence=XYX  RotationSequenceAngles=[0 0 0]  RotationSequenceAnglesUnits=deg  RotationMatrix=[1 0 0; 0 1 0; 0 0 1]
  Input Revolute Joint : sm_lib/Joints/Revolute Joint  SenseConstraintForce=off  SenseConstraintForceX=off  SenseConstraintForceY=off  SenseConstraintForceZ=off  SenseConstraintTorque=off  SenseConstraintTorqueX=off  SenseConstraintTorqueY=off  SenseConstraintTorqueZ=off  SenseTotalForce=off  SenseTotalForceX=off  SenseTotalForceY=off  SenseTotalForceZ=off  SenseTotalTorque=off  SenseTotalTorqueX=off  SenseTotalTorqueY=off  SenseTotalTorqueZ=off  CompositeWrenchDir=FollowerOnBase  CompositeWrenchFrame=BaseFrame  EquilibriumPosition=0  EquilibriumPositionUnits=rad  SpringStiffness=0  SpringStiffnessUnits=N*m/rad  DampingCoefficient=0  DampingCoefficientUnits=N*m/(rad/s)  TorqueActuationMode=InputTorque  MotionActuationMode=ComputedMotion  SensePosition=off  SenseVelocity=on  SenseAcceleration=off  SenseTorqueForce=off  PositionTargetSpecify=off  PositionTargetPriority=High  PositionTargetValue=0  PositionTargetValueUnits=deg  VelocityTargetSpecify=off  VelocityTargetPriority=High  VelocityTargetValue=0  VelocityTargetValueUnits=rad/s
  MATLAB Function : MATLAB Function  TreatAsAtomicUnit=on
  Output Revolute Joint : sm_lib/Joints/Revolute Joint  SenseConstraintForce=off  SenseConstraintForceX=off  SenseConstraintForceY=off  SenseConstraintForceZ=off  SenseConstraintTorque=off  SenseConstraintTorqueX=off  SenseConstraintTorqueY=off  SenseConstraintTorqueZ=off  SenseTotalForce=off  SenseTotalForceX=off  SenseTotalForceY=off  SenseTotalForceZ=off  SenseTotalTorque=off  SenseTotalTorqueX=off  SenseTotalTorqueY=off  SenseTotalTorqueZ=off  CompositeWrenchDir=FollowerOnBase  CompositeWrenchFrame=BaseFrame  EquilibriumPosition=0  EquilibriumPositionUnits=rad  SpringStiffness=0  SpringStiffnessUnits=N*m/rad  DampingCoefficient=1  DampingCoefficientUnits=N*m/(rad/s)  TorqueActuationMode=NoTorque  MotionActuationMode=ComputedMotion  SensePosition=on  SenseVelocity=on  SenseAcceleration=off  SenseTorqueForce=off  PositionTargetSpecify=on  PositionTargetPriority=High  PositionTargetValue=initialPosition  PositionTargetValueUnits=rad  VelocityTargetSpecify=on  VelocityTargetPriority=High  VelocityTargetValue=initialVelocity  VelocityTargetValueUnits=rad/s
  PS-Simulink Converter : nesl_utility/PS-Simulink Converter  PhysicalDomain=network_engine_domain  SubClassName=ps_output  LeftPortType=input  RightPortType=output  PseudoPeriodic=off  Frequencies=[]  Unit=rad  AffineConversion=off
  PS-Simulink Converter1 : nesl_utility/PS-Simulink Converter  PhysicalDomain=network_engine_domain  SubClassName=ps_output  LeftPortType=input  RightPortType=output  PseudoPeriodic=off  Frequencies=[]  Unit=rad/s  AffineConversion=off
  PS-Simulink Converter2 : nesl_utility/PS-Simulink Converter  PhysicalDomain=network_engine_domain  SubClassName=ps_output  LeftPortType=input  RightPortType=output  PseudoPeriodic=off  Frequencies=[]  Unit=rad/s  AffineConversion=off
  Quantizer : Quantizer  QuantizationInterval=(2*pi)/(encoderResolution*gearRatio)
  Rate Transition : RateTransition  Deterministic=off  InitialCondition=initialPosition  OutPortSampleTimeOpt=Inherit
  Rate Transition1 : RateTransition  Deterministic=off  InitialCondition=initialPosition  OutPortSampleTimeOpt=Inherit
  Rotor Solid : sm_lib/Body Elements/Solid  InertiaType=Custom  Mass=0  MassUnits=kg  CenterOfMass=[0; 0; 0]  CenterOfMassUnits=m  MomentsOfInertia=[0; 0; rotorInertia]  MomentsOfInertiaUnits=kg*m^2  ProductsOfInertia=[0; 0; 0]  ProductsOfInertiaUnits=kg*m^2  DensityBased=on  Density=1000  DensityUnits=kg/m^3  DoExposeReferenceFrame=on  SerializedFrames=<Frames/>  GraphicType=None  MarkerShape=Sphere  MarkerSize=10  GraphicVisPropType=SimpleVisualProperties  GraphicDiffuseColor=[0.5 0.5 0.5]  GraphicSpecularColor=[0.5 0.5 0.5 1.0]  GraphicAmbientColor=[0.15 0.15 0.15 1.0]  GraphicEmissiveColor=[0.0 0.0 0.0 1.0]  GraphicShininess=75  GraphicOpacity=1.0  GeometryShape=Cylinder  RectangleSize=[1 1]  RectangleSizeUnits=m  BrickDimensions=[1 1 1]  BrickDimensionUnits=m  CylinderRadius=1  CylinderRadiusUnits=m  CylinderLength=1  CylinderLengthUnits=m  SphereRadius=1  SphereRadiusUnits=m  EllipsoidRadii=[1 1 1]  EllipsoidRadiiUnits=m  ExtrusionCrossSection=[1 1; -1 1; -1 -1; 1 -1]  ExtrusionCrossSectionUnits=m  ExtrusionLength=1  ExtrusionLengthUnits=m  PolygonNumSides=3  PolygonOuterRadius=1  PolygonOuterRadiusUnits=m  ExtGeomFileType=STEP  ExtGeomFileUnits=m  RevolutionCrossSection=[1 1; 1 -1; 2 -1; 2 1]  RevolutionCrossSectionUnits=m  RevolutionExtent=Full  RevolutionAngle=180  RevolutionAngleUnits=deg
  Simulink-PS Converter : nesl_utility/Simulink-PS Converter  PhysicalDomain=network_engine_domain  SubClassName=ps_input  LeftPortType=input  RightPortType=output  PseudoPeriodic=off  Frequencies=[]  NoiseDistribution=none  NoiseParameters=[]  Unit=N*m  AffineConversion=off  FilteringAndDerivatives=zero  SimscapeFilterOrder=1  InputFilterTimeConstant=0.001  UdotUserProvided=1
  Target Torque Scaling : Gain  Gain=-1/gearRatio
  Base : PMIOPort  Port=1  Side=Left
  Follower : PMIOPort  Port=2  Side=Right
  Bus Element Out3 : Outport  PortName=OutBus  Element=statusWord
  Bus Element Out : Outport  PortName=OutBus  Element=position
  Bus Element Out4 : Outport  PortName=OutBus  Element=velocity
  Bus Element Out2 : Outport  PortName=OutBus  Element=torque
  Bus Element Out1 : Outport  PortName=OutBus  Element=driveTemperature
  Bus Element Out5 : Outport  PortName=OutBus  Element=dcLinkVoltage
  Bus Element Out6 : Outport  PortName=OutBus  Element=torqueLimit
  Bus Element Out7 : Outport  PortName=OutBus  Element=gearRatio
  Pos : Outport  Port=2
  vel : Outport  Port=3
  wires:
  PS-Simulink Converter2/1 -> vel/1, Rate Transition1/1
  Rate Transition1/1 -> Bus Element Out4/1
  Constant5/1 -> Bus Element Out7/1
  Actual Torque Scaling/1 -> Bus Element Out2/1
  Constant4/1 -> Bus Element Out6/1
  Constant3/1 -> Bus Element Out5/1
  Constant1/1 -> Bus Element Out1/1
  Constant2/1 -> Bus Element Out3/1
  Target Torque Scaling/1 -> MATLAB Function/2("torque ")
  PS-Simulink Converter1/1 -> MATLAB Function/1(speed)
  MATLAB Function/1(torque) -> Simulink-PS Converter/1, Actual Torque Scaling/1
  Bus Element In/1 -> Target Torque Scaling/1
  Quantizer/1 -> Bus Element Out/1
  PS-Simulink Converter/1 -> Pos/1, Rate Transition/1
  Rate Transition/1 -> Quantizer/1
  connections:
  Output Revolute Joint/RConn3 -- PS-Simulink Converter2/LConn1
  Input Revolute Joint/LConn1 -- Base/RConn1 -- Gear Constraint Offset/LConn1
  Simulink-PS Converter/RConn1 -- Input Revolute Joint/LConn2
  PS-Simulink Converter1/LConn1 -- Input Revolute Joint/RConn2
  Rotor Solid/RConn1 -- Gear Constraint/LConn1 -- Input Revolute Joint/RConn1
  Output Revolute Joint/RConn1 -- Follower/RConn1 -- Gear Constraint/RConn1
  Output Revolute Joint/LConn1 -- Gear Constraint Offset/RConn1
  Output Revolute Joint/RConn2 -- PS-Simulink Converter/LConn1
